simulink model "Trial_Estimator"  (R2017b)
settings: Solver=FixedStepDiscrete  StartTime=0.0  StopTime=25  FixedStep=0.01  RelTol=1e-3
undefined symbols (not defined in the file or in its folder): bf, br, ca, J, lf, lr, mv, rho
libraries: simulink x3
settings Model: Creator=ashwin.ramanujam  LastModifiedBy=gandh

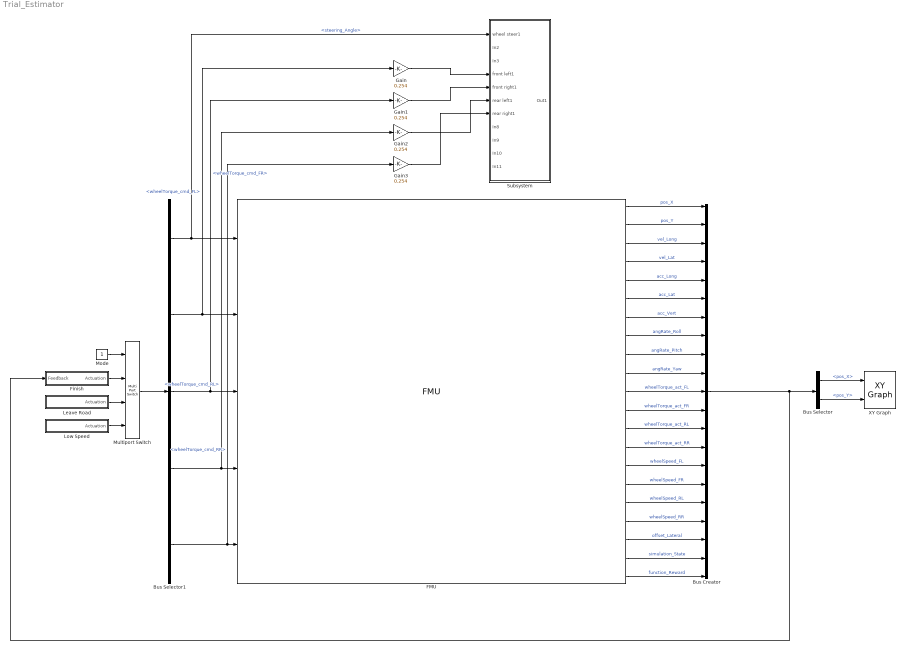
== system Trial_Estimator ==
  Bus Creator : BusCreator  Inputs=21
  Bus Selector : BusSelector  OutputSignals=pos_X,pos_Y
  Bus Selector1 : BusSelector  OutputSignals=steering_Angle,wheelTorque_cmd_FL,wheelTorque_cmd_FR,wheelTorque_cmd_RL,wheelTorque_cmd_RR
  FMU : FMU  FMUName=MED2018_VehicleModel.fmu  FMUDebugLogging=on  FMUMode=CoSimulation  FMUSampleTime=-1  mask(MED2018.VehicleModel [Co-Simulation, v2.0]){}
      mask Display:
      | if (exist([Simulink.fileGenControl('get','CacheFolder') '\slprj\_fmu\ebcf20e87c592f03d69f3ad471d74313\MED2018_VehicleModel\model.png'],'file'))
      |     image([Simulink.fileGenControl('get','CacheFolder') '\slprj\_fmu\ebcf20e87c592f03d69f3ad471d74313\MED2018_VehicleModel\model.png']);
      |     text(0.03, 0.97, 'MED2018.VehicleModel', 'horizontalAlignment', 'left', 'verticalAlignment', 'top');
      | else
      |     disp('MED2018.VehicleModel');
      | end
      | port_label('output',1,'pos_X');
      | port_label('output',2,'pos_Y');
      | port_label('output',3,'vel_Long');
      | port_label('output',4,'vel_Lat');
      | port_label('output',5,'acc_Long');
      | port_label('output',6,'acc_Lat');
      | port_label('output',7,'acc_Vert');
      | port_label('output',8,'angRate_Roll');
      | port_label('output',9,'angRate_Pitch');
      | port_label('output',10,'angRate_Yaw');
      | port_label('output',11,'wheellTorque_act_FL');
      | port_label('output',12,'wheelTorque_act_FR');
      | port_label('output',13,'wheelTorque_act_RL');
      | port_label('output',14,'wheelTorque_act_RR');
      | port_label('output',15,'wheelSpeed_FL');
      | port_label('output',16,'wheelSpeed_FR');
      | port_label('output',17,'wheelSpeed_RL');
      | port_label('output',18,'wheelSpeed_RR');
      | port_label('output',19,'offset_Lateral');
      | port_label('output',20,'simulation_State');
      | port_label('output',21,'function_Reward');
      | port_label('input',1,'steering_Angle');
      | port_label('input',2,'wheelTorque_cmd_FL');
      | port_label('input',3,'wheelTorque_cmd_FR');
      | port_label('input',4,'wheelTorque_cmd_RL');
      | port_label('input',5,'wheelTorque_cmd_RR');
  Finish : Subsystem
  Gain{,1..3} (4 alike) : Gain  Gain=0.254
  Leave Road : Subsystem
  Low Speed : Subsystem
  Mode : Constant
  Multiport Switch : MultiPortSwitch
  Subsystem : Subsystem
  XY Graph : simulink/Sinks/XY Graph  xmin=-1  xmax=110  ymin=-1  ymax=180  st=-1
  wires:
  Multiport Switch/1 -> Bus Selector1/1
  Finish/1(Actuation) -> Multiport Switch/2
  Mode/1 -> Multiport Switch/1
  Bus Selector1/1 -> Subsystem/1(wheel steer1), FMU/1  "<steering_Angle>"
  Bus Selector1/2 -> Gain/1, FMU/2  "<wheelTorque_cmd_FL>"
  Bus Selector1/3 -> Gain1/1, FMU/3  "<wheelTorque_cmd_FR>"
  Bus Selector1/4 -> Gain2/1, FMU/4  "<wheelTorque_cmd_RL>"
  Bus Selector1/5 -> Gain3/1, FMU/5  "<wheelTorque_cmd_RR>"
  FMU/1 -> Bus Creator/1  "pos_X"
  FMU/2 -> Bus Creator/2  "pos_Y"
  FMU/3 -> Bus Creator/3  "vel_Long"
  FMU/4 -> Bus Creator/4  "vel_Lat"
  FMU/5 -> Bus Creator/5  "acc_Long"
  FMU/6 -> Bus Creator/6  "acc_Lat"
  FMU/7 -> Bus Creator/7  "acc_Vert"
  FMU/8 -> Bus Creator/8  "angRate_Roll"
  FMU/9 -> Bus Creator/9  "angRate_Pitch"
  FMU/10 -> Bus Creator/10  "angRate_Yaw"
  FMU/11 -> Bus Creator/11  "wheelTorque_act_FL"
  FMU/12 -> Bus Creator/12  "wheelTorque_act_FR"
  FMU/13 -> Bus Creator/13  "wheelTorque_act_RL"
  FMU/14 -> Bus Creator/14  "wheelTorque_act_RR"
  FMU/15 -> Bus Creator/15  "wheelSpeed_FL"
  FMU/16 -> Bus Creator/16  "wheelSpeed_FR"
  FMU/17 -> Bus Creator/17  "wheelSpeed_RL"
  FMU/18 -> Bus Creator/18  "wheelSpeed_RR"
  FMU/19 -> Bus Creator/19  "offset_Lateral"
  FMU/20 -> Bus Creator/20  "simulation_State"
  FMU/21 -> Bus Creator/21  "function_Reward"
  Bus Selector/1 -> XY Graph/1  "<pos_X>"
  Bus Selector/2 -> XY Graph/2  "<pos_Y>"
  Leave Road/1(Actuation) -> Multiport Switch/3
  Low Speed/1(Actuation) -> Multiport Switch/4
  Bus Creator/1 -> Finish/1(Feedback), Bus Selector/1
  Gain/1 -> Subsystem/4(front left1)
  Gain1/1 -> Subsystem/5(front right1)
  Gain2/1 -> Subsystem/6(rear left1)
  Gain3/1 -> Subsystem/7(rear right1)

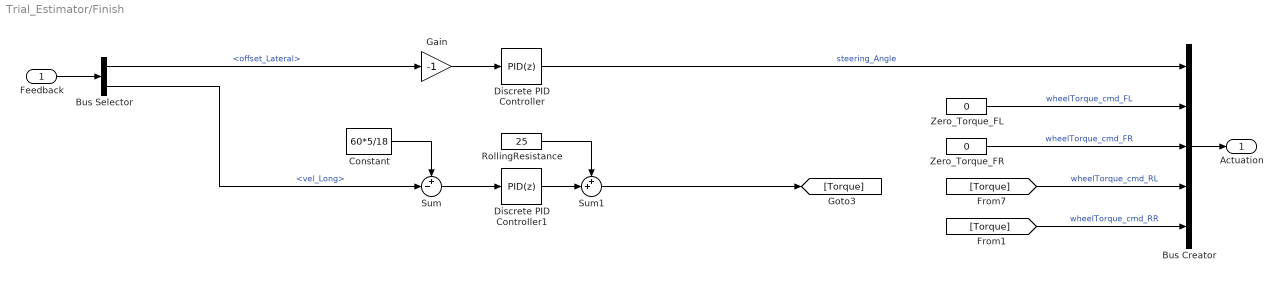
== system Trial_Estimator/Finish ==
  Feedback : Inport
  Bus Creator : BusCreator  Inputs=5
  Bus Selector : BusSelector  OutputSignals=offset_Lateral,vel_Long
  Constant : Constant  Value=60*5/18
  Discrete PID Controller : simulink/Continuous/PID Controller  Controller=PID  TimeDomain=Discrete-time  SampleTime=-1  IntegratorMethod=Forward Euler  FilterMethod=Forward Euler  Form=Parallel  UseFilter=off  ControllerParametersSource=internal  P=1  I=0  D=1  N=100  InitialConditionSource=internal  InitialConditionForIntegrator=0  InitialConditionForFilter=0  ExternalReset=none  LimitOutput=off  UpperSaturationLimit=inf  LowerSaturationLimit=-inf  LinearizeAsGain=off  AntiWindupMode=none  Kb=1  TrackingMode=off  Kt=1  PParamMin=[]  PParamMax=[]  IParamMin=[]  IParamMax=[]  DParamMin=[]  DParamMax=[]  NParamMin=[]  NParamMax=[]  KbParamMin=[]  KbParamMax=[]  KtParamMin=[]  KtParamMax=[]  POutMin=[]  POutMax=[]  IOutMin=[]  IOutMax=[]  DOutMin=[]  DOutMax=[]  NOutMin=[]  NOutMax=[]  KbOutMin=[]  KbOutMax=[]  KtOutMin=[]  KtOutMax=[]  IntegratorOutMin=[]  IntegratorOutMax=[]  FilterOutMin=[]  FilterOutMax=[]  SumOutMin=[]  SumOutMax=[]  SumI1OutMin=[]  SumI1OutMax=[]  SumI2OutMin=[]  SumI2OutMax=[]  SumI3OutMin=[]  SumI3OutMax=[]  SumDOutMin=[]  SumDOutMax=[]  SaturationOutMin=[]  SaturationOutMax=[]  IntegratorContinuousStateAttributes=''  IntegratorStateMustResolveToSignalObject=off  IntegratorRTWStateStorageClass=Auto  FilterContinuousStateAttributes=''  FilterStateMustResolveToSignalObject=off  FilterRTWStateStorageClass=Auto  DifferentiatorICPrevScaledInput=0  DifferentiatorOutMin=[]  DifferentiatorOutMax=[]  InitialConditionSetting=State (most efficient)  FilterDiffOutCoefMin=[]  FilterDiffOutCoefMax=[]  SumDenOutMin=[]  SumDenOutMax=[]  SumNumOutMin=[]  SumNumOutMax=[]  ReciprocalOutMin=[]  ReciprocalOutMax=[]  DivideOutMin=[]  DivideOutMax=[]  TunerSelectOption=Transfer Function Based (PID Tuner App)
  Discrete PID Controller1 : simulink/Continuous/PID Controller  Controller=PID  TimeDomain=Discrete-time  SampleTime=-1  IntegratorMethod=Forward Euler  FilterMethod=Forward Euler  Form=Parallel  UseFilter=on  ControllerParametersSource=internal  P=100  I=0  D=0.1  N=100  InitialConditionSource=internal  InitialConditionForIntegrator=0  InitialConditionForFilter=0  ExternalReset=none  LimitOutput=off  UpperSaturationLimit=inf  LowerSaturationLimit=-inf  LinearizeAsGain=off  AntiWindupMode=none  Kb=1  TrackingMode=off  Kt=1  PParamMin=[]  PParamMax=[]  IParamMin=[]  IParamMax=[]  DParamMin=[]  DParamMax=[]  NParamMin=[]  NParamMax=[]  KbParamMin=[]  KbParamMax=[]  KtParamMin=[]  KtParamMax=[]  POutMin=[]  POutMax=[]  IOutMin=[]  IOutMax=[]  DOutMin=[]  DOutMax=[]  NOutMin=[]  NOutMax=[]  KbOutMin=[]  KbOutMax=[]  KtOutMin=[]  KtOutMax=[]  IntegratorOutMin=[]  IntegratorOutMax=[]  FilterOutMin=[]  FilterOutMax=[]  SumOutMin=[]  SumOutMax=[]  SumI1OutMin=[]  SumI1OutMax=[]  SumI2OutMin=[]  SumI2OutMax=[]  SumI3OutMin=[]  SumI3OutMax=[]  SumDOutMin=[]  SumDOutMax=[]  SaturationOutMin=[]  SaturationOutMax=[]  IntegratorContinuousStateAttributes=''  IntegratorStateMustResolveToSignalObject=off  IntegratorRTWStateStorageClass=Auto  FilterContinuousStateAttributes=''  FilterStateMustResolveToSignalObject=off  FilterRTWStateStorageClass=Auto  DifferentiatorICPrevScaledInput=0  DifferentiatorOutMin=[]  DifferentiatorOutMax=[]  InitialConditionSetting=State (most efficient)  FilterDiffOutCoefMin=[]  FilterDiffOutCoefMax=[]  SumDenOutMin=[]  SumDenOutMax=[]  SumNumOutMin=[]  SumNumOutMax=[]  ReciprocalOutMin=[]  ReciprocalOutMax=[]  DivideOutMin=[]  DivideOutMax=[]  TunerSelectOption=Transfer Function Based (PID Tuner App)
  Gain : Gain  Gain=-1
  RollingResistance : Constant  Value=25
  Sum : Sum  Inputs=+-|
  Sum1 : Sum  Inputs=++|
  Zero_Torque_FL : Constant  Value=0
  Zero_Torque_FR : Constant  Value=0
  Actuation : Outport
  wires:
  Bus Creator/1 -> Actuation/1
  Gain/1 -> Discrete PID Controller/1
  Sum/1 -> Discrete PID Controller1/1
  Feedback/1 -> Bus Selector/1
  Sum1/1 -> [Torque]
  Bus Selector/2 -> Sum/2  "<vel_Long>"
  Constant/1 -> Sum/1
  Bus Selector/1 -> Gain/1  "<offset_Lateral>"
  Discrete PID Controller/1 -> Bus Creator/1  "steering_Angle"
  Discrete PID Controller1/1 -> Sum1/2
  RollingResistance/1 -> Sum1/1
  Zero_Torque_FL/1 -> Bus Creator/2  "wheelTorque_cmd_FL"
  [Torque] -> Bus Creator/4  "wheelTorque_cmd_RL"
  Zero_Torque_FR/1 -> Bus Creator/3  "wheelTorque_cmd_FR"
  [Torque] -> Bus Creator/5  "wheelTorque_cmd_RR"

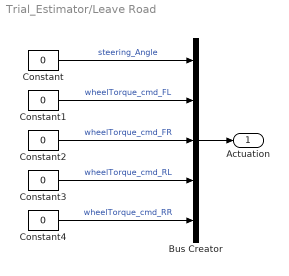
== system Trial_Estimator/Leave Road ==
  Bus Creator : BusCreator  Inputs=5
  Constant{,1..4} (5 alike) : Constant  Value=0
  Actuation : Outport
  wires:
  Constant4/1 -> Bus Creator/5  "wheelTorque_cmd_RR"
  Constant1/1 -> Bus Creator/2  "wheelTorque_cmd_FL"
  Constant3/1 -> Bus Creator/4  "wheelTorque_cmd_RL"
  Constant/1 -> Bus Creator/1  "steering_Angle"
  Constant2/1 -> Bus Creator/3  "wheelTorque_cmd_FR"
  Bus Creator/1 -> Actuation/1

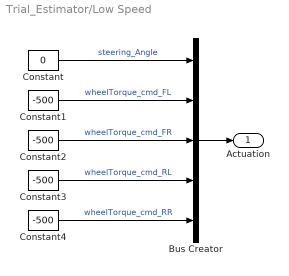
== system Trial_Estimator/Low Speed ==
  Bus Creator : BusCreator  Inputs=5
  Constant : Constant  Value=0
  Constant{1..4} (4 alike) : Constant  Value=-500
  Actuation : Outport
  wires:
  Bus Creator/1 -> Actuation/1
  Constant3/1 -> Bus Creator/4  "wheelTorque_cmd_RL"
  Constant1/1 -> Bus Creator/2  "wheelTorque_cmd_FL"
  Constant/1 -> Bus Creator/1  "steering_Angle"
  Constant4/1 -> Bus Creator/5  "wheelTorque_cmd_RR"
  Constant2/1 -> Bus Creator/3  "wheelTorque_cmd_FR"

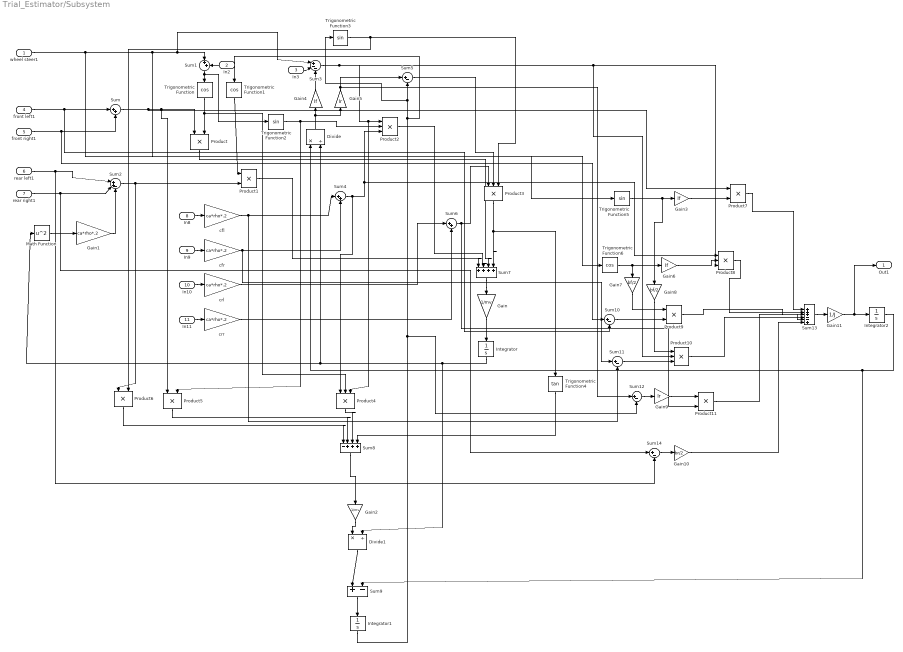
== system Trial_Estimator/Subsystem ==
  wheel steer1 : Inport
  In2 : Inport  Port=2
  In3 : Inport  Port=3
  front left1 : Inport  Port=4
  front right1 : Inport  Port=5
  rear left1 : Inport  Port=6
  rear right1 : Inport  Port=7
  In8 : Inport  Port=8
  In9 : Inport  Port=9
  In10 : Inport  Port=10
  In11 : Inport  Port=11
  Divide : Product  Inputs=*/
  Divide1 : Product  Inputs=*/
  Gain : Gain  Gain=1/mv
  Gain1 : Gain  Gain=ca*rho*.2
  Gain10 : Gain  Gain=br/2
  Gain11 : Gain  Gain=1/J
  Gain2 : Gain  Gain=1/mv
  Gain3 : Gain  Gain=lf
  Gain4 : Gain  Gain=lf
  Gain5 : Gain  Gain=lr
  Gain6 : Gain  Gain=lf
  Gain7 : Gain  Gain=bf/2
  Gain8 : Gain  Gain=bf/2
  Gain9 : Gain  Gain=lr
  Integrator : Integrator
  Integrator1 : Integrator
  Integrator2 : Integrator
  Math Function : Math  Operator=square  SaturateOnIntegerOverflow=on
  Product{,1,5..7,9,11} (7 alike) : Product
  Product{2..4,8,10} (5 alike) : Product  Inputs=3
  Sum{,1,4,6} (4 alike) : Sum  Inputs=|++
  Sum{5,9..12,14} (6 alike) : Sum  Inputs=|+-
  Sum13 : Sum  Inputs=|+++--+
  Sum2 : Sum  Inputs=|++-
  Sum3 : Sum  Inputs=|+--
  Sum7 : Sum  Inputs=|++++
  Sum8 : Sum  Inputs=|-+++
  Trigonometric Function : Trigonometry  Operator=cos
  Trigonometric Function1 : Trigonometry  Operator=cos
  Trigonometric Function2 : Trigonometry
  Trigonometric Function3 : Trigonometry
  Trigonometric Function4 : Trigonometry  Operator=tan
  Trigonometric Function5 : Trigonometry
  Trigonometric Function6 : Trigonometry  Operator=cos
  cfl : Gain  Gain=ca*rho*.2
  cfr : Gain  Gain=ca*rho*.2
  crl : Gain  Gain=ca*rho*.2
  crr : Gain  Gain=ca*rho*.2
  Out1 : Outport
  wires:
  Integrator1/1 -> Sum12/2, Trigonometric Function1/1, Trigonometric Function3/1, Sum5/2
  Sum9/1 -> Integrator1/1
  Sum2/1 -> Product6/1, Product1/2
  In8/1 -> cfl/1
  In10/1 -> crl/1
  front right1/1 -> Sum10/1, Sum/2
  Sum/1 -> Product7/1, Product5/1, Product/1
  Gain6/1 -> Product8/2
  Divide/1 -> Gain5/1, Gain4/1
  crr/1 -> Sum6/2
  Gain7/1 -> Product9/1
  Trigonometric Function6/1 -> Gain6/1, Gain7/1
  In2/1 -> Sum1/2
  In3/1 -> Sum3/2
  Product7/1 -> Sum13/1
  Math Function/1 -> Gain1/1
  Gain11/1 -> Out1/1, Integrator2/1
  Sum7/1 -> Gain/1
  In11/1 -> crr/1
  Sum4/1 -> Product4/1, Product8/1, Product2/3
  Gain10/1 -> Sum13/6
  Gain3/1 -> Product7/2
  Trigonometric Function5/1 -> Gain8/1, Gain3/1
  Trigonometric Function4/1 -> Sum8/4
  Product8/1 -> Sum13/2
  Integrator2/1 -> Sum9/2, Divide/1
  Divide1/1 -> Sum9/1
  Product4/1 -> Sum8/3
  crl/1 -> Sum6/1
  Sum14/1 -> Gain10/1
  Sum12/1 -> Gain9/1
  Product9/1 -> Sum13/3
  rear left1/1 -> Sum14/2, Sum2/1
  Sum13/1 -> Gain11/1
  Product/1 -> Sum7/3
  Product2/1 -> Sum7/2
  Sum1/1 -> Trigonometric Function2/1, Trigonometric Function/1
  Sum5/1 -> Product3/2
  Gain8/1 -> Product10/1
  Product3/1 -> Trigonometric Function4/1, Sum7/4
  Sum11/1 -> Product10/3
  Gain4/1 -> Sum3/3
  Gain9/1 -> Product11/1
  Gain1/1 -> Sum2/3
  Sum6/1 -> Product11/2, Product3/1
  Product1/1 -> Sum7/1
  Product5/1 -> Sum8/2
  Product6/1 -> Sum8/1
  Sum10/1 -> Product9/2
  In9/1 -> cfr/1
  Gain5/1 -> Sum12/1, Sum5/1
  Integrator/1 -> Divide1/2, Divide/2, Math Function/1
  Trigonometric Function/1 -> Product4/2, Product/2
  cfl/1 -> Sum11/2, Sum4/1
  Product11/1 -> Sum13/5
  Trigonometric Function2/1 -> Product5/2, Product2/2
  Sum3/1 -> Product10/2, Product8/3, Product4/3, Product2/1
  front left1/1 -> Sum10/2, Sum/1
  cfr/1 -> Sum11/1, Sum4/2
  rear right1/1 -> Sum14/1, Sum2/2
  Gain2/1 -> Divide1/1
  Trigonometric Function3/1 -> Product6/2, Product3/3
  Sum8/1 -> Gain2/1
  Trigonometric Function1/1 -> Product1/1
  Gain/1 -> Integrator/1
  wheel steer1/1 -> Trigonometric Function6/1, Trigonometric Function5/1, Sum3/1, Sum1/1
  Product10/1 -> Sum13/4
